simulink model "baseline_queso_1_1"  (R2021a)
settings: Solver=FixedStepAuto  StartTime=0.0  StopTime=50  FixedStep=framePeriod_s  RelTol=1e-3
undefined symbols (not defined in the file or in its folder): Aircraft, analog, aux, Earth, framePeriod_s, mode, motors_enabled, pwm, sbus, throttle_cmd_prcnt, waypoint_reached, WGS84
libraries: simulink x26, pid_lib x11, aerolibtransform2 x3, simulink_extras x2, aerolibguid x1
(part 1 of 3)
settings Model: Creator=brian  LastModifiedBy=Tuan Luong
settings SolverCC: AlgebraicLoopSolver=TrustRegion
settings OptimizationCC: DefaultParameterBehavior=Inlined  GainParamInheritBuiltInType=on  UseFloatMulNetSlope=on  DefaultUnderspecifiedDataType=single  InlineInvariantSignals=on  PassReuseOutputArgsAs=Individual arguments  ZeroExternalMemoryAtStartup=off  ZeroInternalMemoryAtStartup=off  NoFixptDivByZeroProtection=on  EfficientFloat2IntCast=on  LifeSpan=1  OptimizeBlockOrder=speed  DifferentSizesBufferReuse=on  EfficientTunableParamExpr=on
settings DebuggingCC: ParameterTunabilityLossMsg=error  SFMachineParentedDataDiag=warning
settings HardwareCC: ProdBitPerPointer=32  ProdBitPerSizeT=32  ProdBitPerPtrDiffT=32  ProdLargestAtomicInteger=Long  ProdLargestAtomicFloat=Double  ProdWordSize=32  ProdLongLongMode=on  ProdHWDeviceType=NXP->Cortex-M4
settings ModelReferenceCC: ModelReferenceNumInstancesAllowed=Single
settings SFSimCC: SimParseCustomCode=off  MATLABDynamicMemAlloc=off
settings RTWCC: SystemTargetFile=ert.tlc  GenCodeOnly=on  TemplateMakefile=ert_default_tmf  RTWVerbose=off  Toolchain=Microsoft Visual C++ 2019 v16.0 | nmake (64-bit Windows)  BuildConfiguration=Faster Runs  TargetLang=C++
settings CodeAppCC: ForceParamTrailComments=on  IgnoreCustomStorageClasses=off  OperatorAnnotations=on  SimulinkDataObjDesc=on  SFDataObjDesc=on  CustomSymbolStrGlobalVar=rt$N$M  CustomSymbolStrType=$N$M  CustomSymbolStrFcn=$N$M$F  CustomSymbolStrMacro=$N$M  InsertBlockDesc=on
settings ERTTargetCC: TargetLangStandard=C++03 (ISO)  IncludeMdlTerminateFcn=off  CombineSignalStateStructs=on  SuppressErrorStatus=on  SupportAbsoluteTime=off  CodeInterfacePackaging=C++ class  SupportNonFinite=off  SupportComplex=off  ERTHeaderFileRootName=autocode$E  ERTSourceFileRootName=autocode$E  InlinedParameterPlacement=NonHierarchical  RootIOFormat=Structure reference  ERTCustomFileTemplate=example_file_process.tlc  ERTFilePackagingFormat=Compact  ArrayContainerType=std::array

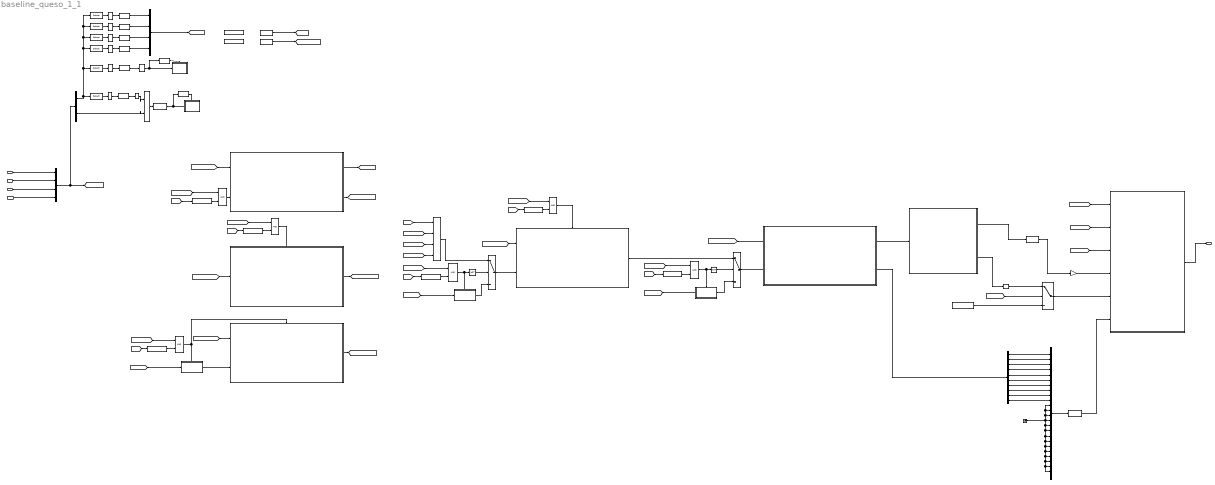
== system baseline_queso_1_1 ==
  System Data : Inport  OutDataTypeStr=Bus: SysData  SampleTime=framePeriod_s  BusOutputAsStruct=on
  Sensor Data : Inport  Port=2  OutDataTypeStr=Bus: SensorData  SampleTime=framePeriod_s  BusOutputAsStruct=on
  Navigation Filter Data : Inport  Port=3  OutDataTypeStr=Bus: NavData  SampleTime=framePeriod_s  BusOutputAsStruct=on
  Telemetry Data : Inport  Port=4  OutDataTypeStr=Bus: TelemData  SampleTime=framePeriod_s  BusOutputAsStruct=on
  ANGLE CONTROLLER : Subsystem
  Bus Creator2 : BusCreator  Inputs=24
  Bus Selector : BusSelector  OutputSignals=Sensor Data.inceptor.ch,Navigation Filter Data.nav_initialized
  Bus Selector1 : BusSelector  OutputSignals=throttle,roll_cc,roll_cmd_rad,roll_rad,pitch_cc,pitch_cmd_rad,pitch_rad,yaw_cc,yaw_rate_cmd_radps,yaw_rate_radps
  Cast To Boolean1 : DataTypeConversion  OutDataTypeStr=boolean
  Cast To Single : DataTypeConversion  OutDataTypeStr=single
  Cast To Single1 : DataTypeConversion  OutDataTypeStr=single
  Compare To Constant : simulink/Logic and Bit Operations/Compare To Constant  relop=>  const=0  OutDataTypeStr=boolean
  Constant : Constant  Value=[0 0 0 0 0 0 0 0]  OutDataTypeStr=single  SampleTime=framePeriod_s
  Data Store Read : DataStoreRead  DataStoreName=cur_mode  SampleTime=framePeriod_s  IndexOptions=Index vector (dialog)  Indices=1  OutputSizes=1
  Data Store Read1 : DataStoreRead  DataStoreName=motor_state  SampleTime=framePeriod_s  IndexOptions=Index vector (dialog)  Indices=1  OutputSizes=1
  Data Type Conversion{,1..5} (6 alike) : DataTypeConversion  OutDataTypeStr=single
  Data Type Conversion6 : DataTypeConversion  OutDataTypeStr=int8  RndMeth=Nearest
  Gain : Gain  Gain=100
  Ground : Ground
  LAND CONTROLLER : Subsystem
  Motor Mixing Algorithm : Subsystem
  Multiport Switch : MultiPortSwitch  DataPortOrder=Specify indices  DataPortIndices={2,3,4}  DiagnosticForDefault=None
  NOT : Logic  Operator=NOT  IconShape=distinctive  AllPortsSameDT=off  OutDataTypeStr=boolean
  NOT1 : Logic  Operator=NOT  IconShape=distinctive  AllPortsSameDT=off  OutDataTypeStr=boolean
  POS_HOLD CONTROLLER : Subsystem
  Pos_Hold_input_conversion : Subsystem
  Pos_Hold_input_conversion2 : Subsystem
  RTL CONTROLLER : Subsystem
  Reshape : Reshape
  Stab_input_conversion : Subsystem
  Switch : Switch  Criteria=u2 > Threshold  Threshold=0.5
  Switch1 : Switch  Criteria=u2 > Threshold  Threshold=0.5
  To VMS Data : Subsystem
  WAYPOINT CONTROLLER : Subsystem
  cmd_bus : BusCreator  Inputs=4
  compare_to_land : simulink/Logic and Bit Operations/Compare To Constant  relop===  const=4  OutDataTypeStr=boolean
  compare_to_pos_hold : simulink/Logic and Bit Operations/Compare To Constant  relop=>  const=0  OutDataTypeStr=boolean
  compare_to_rtl : simulink/Logic and Bit Operations/Compare To Constant  relop===  const=3  OutDataTypeStr=boolean
  compare_to_stab : simulink/Logic and Bit Operations/Compare To Constant  relop=<=  const=0  OutDataTypeStr=boolean
  compare_to_stab1 : simulink/Logic and Bit Operations/Compare To Constant  relop===  const=1  OutDataTypeStr=boolean
  compare_to_wp : simulink/Logic and Bit Operations/Compare To Constant  relop===  const=2  OutDataTypeStr=boolean
  data_sys_bus : BusCreator  Inputs=4
  detect_manual_arming : simulink/Logic and Bit Operations/Detect Change  vinit=0  OutDataTypeStr=boolean
  detect_mode_change : simulink/Logic and Bit Operations/Detect Change  vinit=0  OutDataTypeStr=boolean
  flight_mode : DataStoreMemory  DataStoreName=cur_mode  ReadBeforeWriteMsg=warning  WriteAfterWriteMsg=warning  WriteAfterReadMsg=warning  ShowAdditionalParam=off  OutDataTypeStr=int8
  manual_arming : Subsystem
  manual_mode_selection : Subsystem
  mode_norm : Polyval  Coefs=Aircraft.Inceptor.coef_3
  motor_armed AND mode_{0..5} (6 alike) : Logic  IconShape=distinctive  AllPortsSameDT=off  OutDataTypeStr=boolean
  motor_state : DataStoreMemory  DataStoreName=motor_state  ReadBeforeWriteMsg=warning  WriteAfterWriteMsg=warning  WriteAfterReadMsg=warning  ShowAdditionalParam=off  OutDataTypeStr=boolean
  nav_init AND motor_enable : Logic  IconShape=distinctive  AllPortsSameDT=off  OutDataTypeStr=boolean
  pitch_norm : Polyval  Coefs=Aircraft.Inceptor.coef_2
  roll_norm : Polyval  Coefs=Aircraft.Inceptor.coef_2
  select_mode : Selector  IndexOptions=Index vector (dialog)  Indices=Aircraft.Inceptor.mode0  OutputSizes=1
  select_pitch : Selector  IndexOptions=Index vector (dialog)  Indices=Aircraft.Inceptor.pitch  OutputSizes=1
  select_roll : Selector  IndexOptions=Index vector (dialog)  Indices=Aircraft.Inceptor.roll  OutputSizes=1
  select_throttle : Selector  IndexOptions=Index vector (dialog)  Indices=Aircraft.Inceptor.throttle  OutputSizes=1
  select_throttle_en : Selector  IndexOptions=Index vector (dialog)  Indices=Aircraft.Inceptor.throttle_en  OutputSizes=1
  select_yaw : Selector  IndexOptions=Index vector (dialog)  Indices=Aircraft.Inceptor.yaw  OutputSizes=1
  switch_motor_out : Switch  Criteria=u2 > Threshold
  throttle_en_norm : Polyval  Coefs=Aircraft.Inceptor.coef_2
  throttle_norm : Polyval  Coefs=Aircraft.Inceptor.coef_1
  yaw_norm : Polyval  Coefs=Aircraft.Inceptor.coef_2
  VmsData : Outport  OutDataTypeStr=Bus: VmsData  SampleTime=framePeriod_s  BusOutputAsStruct=on
  wires:
  Telemetry Data/1 -> data_sys_bus/3  "Telemetry Data"
  System Data/1 -> data_sys_bus/4  "System Data"
  Sensor Data/1 -> data_sys_bus/1  "Sensor Data"
  Navigation Filter Data/1 -> data_sys_bus/2  "Navigation Filter Data"
  To VMS Data/1(VmsData) -> VmsData/1  "VmsData"
  [arm_state] -> motor_armed AND mode_0/1
  [arm_state] -> motor_armed AND mode_1/1
  [Mode] -> compare_to_pos_hold/1
  compare_to_pos_hold/1 -> motor_armed AND mode_1/2
  Motor Mixing Algorithm/2(PWM) -> Reshape/1
  switch_motor_out/1 -> To VMS Data/5(PWM In)
  [arm_state] -> switch_motor_out/2
  Constant/1 -> switch_motor_out/3
  ANGLE CONTROLLER/1(Command out) -> Motor Mixing Algorithm/1(MMA Bus)
  compare_to_stab/1 -> motor_armed AND mode_0/2
  [Mode] -> compare_to_stab/1
  [Mode] -> To VMS Data/3(Mode in)
  compare_to_wp/1 -> motor_armed AND mode_2/2
  [Mode] -> compare_to_wp/1
  [arm_state] -> motor_armed AND mode_2/1
  Bus Selector/2 -> nav_init AND motor_enable/2  "<nav_initialized>"
  WAYPOINT CONTROLLER/2(wp_reached) -> [waypoint_reached]
  nav_init AND motor_enable/1 -> Cast To Boolean1/1
  [waypoint_reached] -> To VMS Data/2(waypoint_reached)
  [arm_state] -> To VMS Data/1(motors_enabled)
  Motor Mixing Algorithm/1(throttle) -> Cast To Single1/1
  Bus Selector/1 -> select_throttle/1, select_pitch/1, select_roll/1, select_yaw/1, select_mode/1, select_throttle_en/1  "<ch>"
  select_throttle/1 -> Data Type Conversion5/1
  select_pitch/1 -> Data Type Conversion4/1
  select_roll/1 -> Data Type Conversion3/1
  select_yaw/1 -> Data Type Conversion2/1
  select_mode/1 -> Data Type Conversion1/1
  throttle_norm/1 -> cmd_bus/1  "throttle"
  pitch_norm/1 -> cmd_bus/2  "pitch"
  roll_norm/1 -> cmd_bus/3  "roll"
  yaw_norm/1 -> cmd_bus/4  "yaw"
  throttle_en_norm/1 -> Compare To Constant/1  "throttle_en"
  Compare To Constant/1 -> nav_init AND motor_enable/1
  cmd_bus/1 -> [cmd]
  select_throttle_en/1 -> Data Type Conversion/1
  Data Type Conversion/1 -> throttle_en_norm/1
  Data Type Conversion1/1 -> mode_norm/1
  Data Type Conversion2/1 -> yaw_norm/1
  Data Type Conversion3/1 -> roll_norm/1
  Data Type Conversion4/1 -> pitch_norm/1
  Data Type Conversion5/1 -> throttle_norm/1
  mode_norm/1 -> Data Type Conversion6/1  "mode"
  Data Store Read/1 -> [Mode]
  Data Type Conversion6/1 -> manual_mode_selection/1(mode_input), detect_mode_change/1
  detect_mode_change/1 -> manual_mode_selection/Enable
  detect_manual_arming/1 -> manual_arming/Enable
  Cast To Boolean1/1 -> detect_manual_arming/1, manual_arming/1(mode_input)
  Data Store Read1/1 -> [arm_state]
  Pos_Hold_input_conversion2/1(pos_hold_input) -> LAND CONTROLLER/2(Cmd_input)
  compare_to_land/1 -> motor_armed AND mode_4/2
  data_sys_bus/1 -> [sys_input], Bus Selector/1
  [Mode] -> compare_to_land/1
  [arm_state] -> motor_armed AND mode_4/1
  [arm_state] -> motor_armed AND mode_3/1
  motor_armed AND mode_3/1 -> RTL CONTROLLER/Enable
  compare_to_rtl/1 -> motor_armed AND mode_3/2
  [Mode] -> compare_to_rtl/1
  Bus Creator2/1 -> Cast To Single/1
  Gain/1 -> To VMS Data/4(throttle_cmd_prcnt)
  Ground/1 -> Bus Creator2/20, Bus Creator2/21, Bus Creator2/24, Bus Creator2/23, Bus Creator2/22, Bus Creator2/19, Bus Creator2/18, Bus Creator2/17, Bus Creator2/16, Bus Creator2/15, Bus Creator2/11, Bus Creator2/12, Bus Creator2/13, Bus Creator2/14
  Cast To Single/1 -> To VMS Data/6(Aux)
  Cast To Single1/1 -> Gain/1
  [cmd] -> Stab_input_conversion/1(cmd)
  motor_armed AND mode_0/1 -> NOT/1, Stab_input_conversion/Enable
  [sys_input] -> ANGLE CONTROLLER/1(Sys_input)
  Switch/1 -> ANGLE CONTROLLER/2(Cmd_input)
  NOT/1 -> Switch/2
  Stab_input_conversion/1(angle_ctrl_input) -> Switch/3
  [sys_input] -> POS_HOLD CONTROLLER/1(Sys_input)
  motor_armed AND mode_1/1 -> POS_HOLD CONTROLLER/Enable
  [cmd] -> Pos_Hold_input_conversion/1(cmd)
  motor_armed AND mode_5/1 -> Pos_Hold_input_conversion/Enable, NOT1/1
  [Mode] -> compare_to_stab1/1
  compare_to_stab1/1 -> motor_armed AND mode_5/2
  [arm_state] -> motor_armed AND mode_5/1
  NOT1/1 -> Switch1/2
  Switch1/1 -> POS_HOLD CONTROLLER/2(Cmd_input)
  Pos_Hold_input_conversion/1(pos_hold_input) -> Switch1/3
  POS_HOLD CONTROLLER/1(Command out) -> Switch/1
  motor_armed AND mode_2/1 -> WAYPOINT CONTROLLER/2(auto_trigger)
  Multiport Switch/1 -> Switch1/1
  [Mode] -> Multiport Switch/1
  WAYPOINT CONTROLLER/1(wp_command) -> [wp_cmd]
  [wp_cmd] -> Multiport Switch/2
  [sys_input] -> WAYPOINT CONTROLLER/1(Sys_input)
  [sys_input] -> RTL CONTROLLER/1(Sys_input)
  RTL CONTROLLER/1(Command out) -> [rtl_cmd]
  [rtl_cmd] -> Multiport Switch/3
  [sys_input] -> LAND CONTROLLER/1(Sys_input)
  [cmd] -> Pos_Hold_input_conversion2/1(cmd)
  LAND CONTROLLER/1(land_cmd) -> [land_cmd]
  [land_cmd] -> Multiport Switch/4
  motor_armed AND mode_4/1 -> LAND CONTROLLER/Enable, Pos_Hold_input_conversion2/Enable
  ANGLE CONTROLLER/2(inner_loop_log) -> Bus Selector1/1
  Bus Selector1/1 -> Bus Creator2/1  "<throttle>"
  Bus Selector1/2 -> Bus Creator2/2  "<roll_cc>"
  Bus Selector1/3 -> Bus Creator2/3  "<roll_cmd_rad>"
  Bus Selector1/4 -> Bus Creator2/4  "<roll_rad>"
  Bus Selector1/5 -> Bus Creator2/5  "<pitch_cc>"
  Bus Selector1/6 -> Bus Creator2/6  "<pitch_cmd_rad>"
  Bus Selector1/8 -> Bus Creator2/8  "<yaw_cc>"
  Bus Selector1/7 -> Bus Creator2/7  "<pitch_rad>"
  Bus Selector1/9 -> Bus Creator2/9  "<yaw_rate_cmd_radps>"
  Bus Selector1/10 -> Bus Creator2/10  "<yaw_rate_radps>"
  Reshape/1 -> switch_motor_out/1

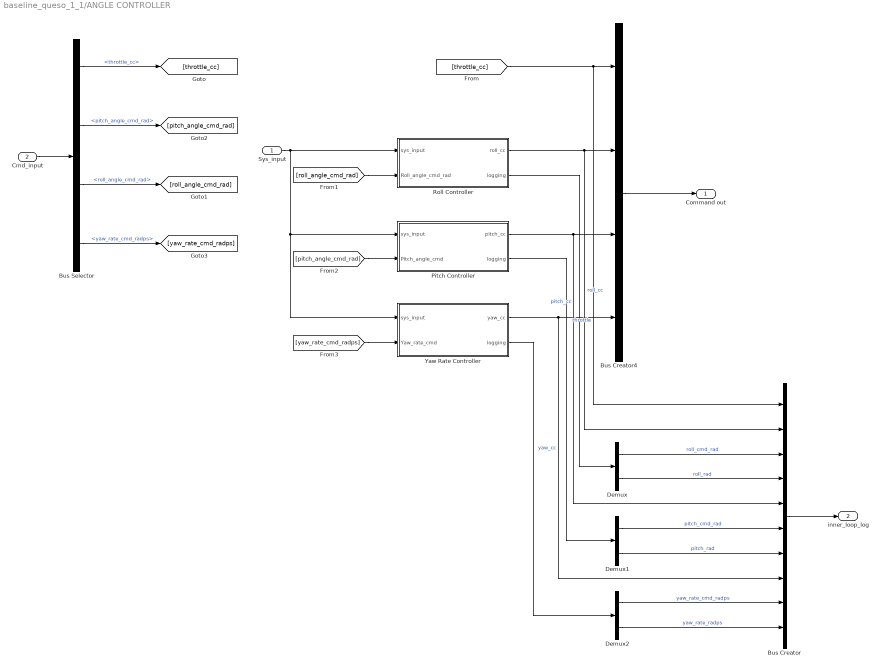
== system baseline_queso_1_1/ANGLE CONTROLLER ==
  Sys_input : Inport
  Cmd_input : Inport  Port=2
  Bus Creator : BusCreator  Inputs=10
  Bus Creator4 : BusCreator  Inputs=4
  Bus Selector : BusSelector  OutputSignals=throttle_cc,pitch_angle_cmd_rad,roll_angle_cmd_rad,yaw_rate_cmd_radps
  Demux : Demux  Outputs=2
  Demux1 : Demux  Outputs=2
  Demux2 : Demux  Outputs=2
  Pitch Controller : Subsystem
  Roll Controller : Subsystem
  Yaw Rate Controller : Subsystem
  Command out : Outport
  inner_loop_log : Outport  Port=2
  wires:
  Bus Creator4/1 -> Command out/1
  Cmd_input/1 -> Bus Selector/1
  Yaw Rate Controller/1(yaw_cc) -> Bus Creator4/4, Bus Creator/8  "yaw_cc"
  Pitch Controller/1(pitch_cc) -> Bus Creator4/3, Bus Creator/5  "pitch_cc"
  Roll Controller/1(roll_cc) -> Bus Creator4/2, Bus Creator/2  "roll_cc"
  Sys_input/1 -> Roll Controller/1(sys_input), Pitch Controller/1(sys_input), Yaw Rate Controller/1(sys_input)
  Bus Selector/1 -> [throttle_cc]  "<throttle_cc>"
  Bus Selector/4 -> [yaw_rate_cmd_radps]  "<yaw_rate_cmd_radps>"
  Bus Selector/2 -> [pitch_angle_cmd_rad]  "<pitch_angle_cmd_rad>"
  Bus Selector/3 -> [roll_angle_cmd_rad]  "<roll_angle_cmd_rad>"
  [throttle_cc] -> Bus Creator/1, Bus Creator4/1  "throttle"
  [roll_angle_cmd_rad] -> Roll Controller/2(Roll_angle_cmd_rad)
  [pitch_angle_cmd_rad] -> Pitch Controller/2(Pitch_angle_cmd)
  [yaw_rate_cmd_radps] -> Yaw Rate Controller/2(Yaw_rate_cmd)
  Demux/1 -> Bus Creator/3  "roll_cmd_rad"
  Demux/2 -> Bus Creator/4  "roll_rad"
  Roll Controller/2(logging) -> Demux/1
  Demux1/1 -> Bus Creator/6  "pitch_cmd_rad"
  Demux1/2 -> Bus Creator/7  "pitch_rad"
  Pitch Controller/2(logging) -> Demux1/1
  Demux2/1 -> Bus Creator/9  "yaw_rate_cmd_radps"
  Demux2/2 -> Bus Creator/10  "yaw_rate_radps"
  Yaw Rate Controller/2(logging) -> Demux2/1
  Bus Creator/1 -> inner_loop_log/1

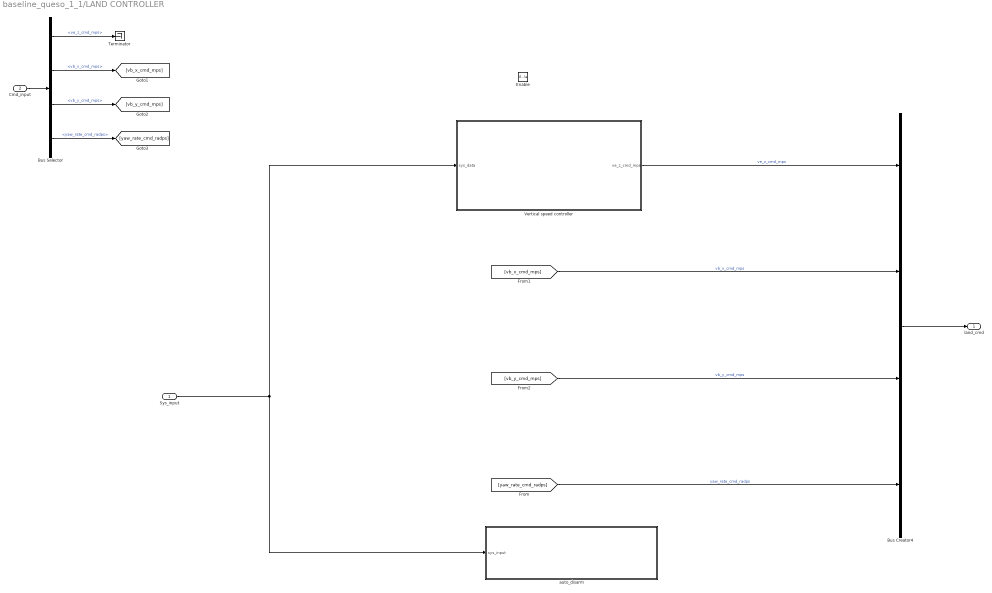
== system baseline_queso_1_1/LAND CONTROLLER ==
  Sys_input : Inport
  Cmd_input : Inport  Port=2
  Enable : EnablePort  PropagateVarSize=During execution
  Bus Creator4 : BusCreator  Inputs=4
  Bus Selector : BusSelector  OutputSignals=ve_z_cmd_mps,vb_x_cmd_mps,vb_y_cmd_mps,yaw_rate_cmd_radps
  Terminator : Terminator
  Vertical speed controller : Subsystem
  auto_disarm : Subsystem
  land_cmd : Outport
  wires:
  Bus Creator4/1 -> land_cmd/1
  Sys_input/1 -> Vertical speed controller/1(sys_data), auto_disarm/1(sys_input)
  Vertical speed controller/1(ve_z_cmd_mps) -> Bus Creator4/1  "ve_z_cmd_mps"
  [vb_x_cmd_mps] -> Bus Creator4/2  "vb_x_cmd_mps"
  [vb_y_cmd_mps] -> Bus Creator4/3  "vb_y_cmd_mps"
  [yaw_rate_cmd_radps] -> Bus Creator4/4  "yaw_rate_cmd_radps"
  Cmd_input/1 -> Bus Selector/1
  Bus Selector/2 -> [vb_x_cmd_mps]  "<vb_x_cmd_mps>"
  Bus Selector/4 -> [yaw_rate_cmd_radps]  "<yaw_rate_cmd_radps>"
  Bus Selector/3 -> [vb_y_cmd_mps]  "<vb_y_cmd_mps>"
  Bus Selector/1 -> Terminator/1  "<ve_z_cmd_mps>"

== system baseline_queso_1_1/Motor Mixing Algorithm ==
  MMA Bus : Inport
  Bus Selector : BusSelector  OutputSignals=throttle,roll_cc,pitch_cc,yaw_cc
  Motor Mix : Constant  Value=Aircraft.Motor.mix  OutDataTypeStr=single  SampleTime=framePeriod_s
  Multiply : Product  Inputs=**  Multiplication=Matrix(*)  OutDataTypeStr=single
  Mux : Mux
  Reshape : Reshape  OutputDimensionality=Column vector (2-D)
  Saturation : Saturate  UpperLimit=3000  LowerLimit=Aircraft.Control.motor_spin_min
  throttle : Outport
  PWM : Outport  Port=2
  wires:
  Mux/1 -> Reshape/1
  MMA Bus/1 -> Bus Selector/1
  Bus Selector/1 -> throttle/1, Mux/1  "<throttle>"
  Bus Selector/2 -> Mux/2  "<roll_cc>"
  Bus Selector/3 -> Mux/3  "<pitch_cc>"
  Bus Selector/4 -> Mux/4  "<yaw_cc>"
  Multiply/1 -> Saturation/1  "Command"
  Saturation/1 -> PWM/1
  Reshape/1 -> Multiply/2
  Motor Mix/1 -> Multiply/1

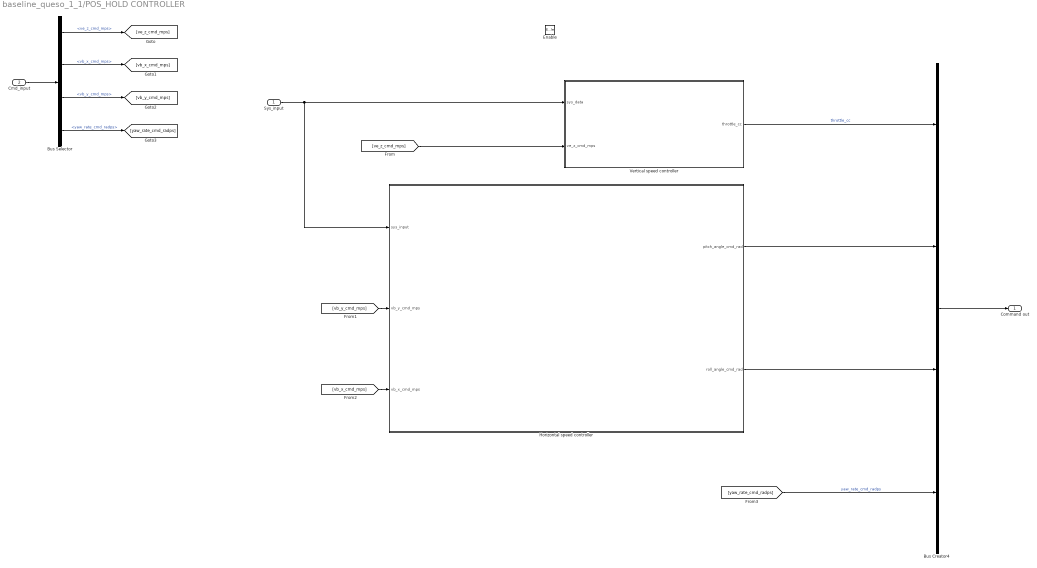
== system baseline_queso_1_1/POS_HOLD CONTROLLER ==
  Sys_input : Inport
  Cmd_input : Inport  Port=2
  Enable : EnablePort  PropagateVarSize=During execution
  Bus Creator4 : BusCreator  Inputs=4
  Bus Selector : BusSelector  OutputSignals=ve_z_cmd_mps,vb_x_cmd_mps,vb_y_cmd_mps,yaw_rate_cmd_radps
  Horizontal speed controller : Subsystem
  Vertical speed controller : Subsystem
  Command out : Outport
  wires:
  Bus Creator4/1 -> Command out/1
  Vertical speed controller/1(throttle_cc) -> Bus Creator4/1  "throttle_cc"
  Sys_input/1 -> Horizontal speed controller/1(sys_input), Vertical speed controller/1(sys_data)
  Cmd_input/1 -> Bus Selector/1
  Bus Selector/1 -> [ve_z_cmd_mps]  "<ve_z_cmd_mps>"
  Bus Selector/2 -> [vb_x_cmd_mps]  "<vb_x_cmd_mps>"
  Bus Selector/3 -> [vb_y_cmd_mps]  "<vb_y_cmd_mps>"
  Bus Selector/4 -> [yaw_rate_cmd_radps]  "<yaw_rate_cmd_radps>"
  [yaw_rate_cmd_radps] -> Bus Creator4/4  "yaw_rate_cmd_radps"
  [ve_z_cmd_mps] -> Vertical speed controller/2(ve_z_cmd_mps)
  [vb_y_cmd_mps] -> Horizontal speed controller/2(vb_y_cmd_mps)
  [vb_x_cmd_mps] -> Horizontal speed controller/3(vb_x_cmd_mps)
  Horizontal speed controller/1(pitch_angle_cmd_rad) -> Bus Creator4/2
  Horizontal speed controller/2(roll_angle_cmd_rad) -> Bus Creator4/3

== system baseline_queso_1_1/Pos_Hold_input_conversion ==
  cmd : Inport
  Enable : EnablePort
  Bus Creator : BusCreator  Inputs=4
  Bus Selector2 : BusSelector  OutputSignals=throttle,pitch,roll,yaw
  Gain1 : Gain  Gain=Aircraft.Control.v_hor_max
  Gain2 : Gain  Gain=Aircraft.Control.v_hor_max
  Gain3 : Gain  Gain=Aircraft.Control.yaw_rate_max
  Throttle Mapper : Subsystem
  pos_hold_input : Outport
  wires:
  Bus Selector2/3 -> Gain2/1  "<roll>"
  Gain2/1 -> Bus Creator/3  "vb_y_cmd_mps"
  Bus Selector2/1 -> Throttle Mapper/1(Throttle)  "<throttle>"
  Bus Selector2/2 -> Gain1/1  "<pitch>"
  Bus Creator/1 -> pos_hold_input/1  "pos_hold_input"
  Bus Selector2/4 -> Gain3/1  "<yaw>"
  Gain1/1 -> Bus Creator/2  "vb_x_cmd_mps"
  Gain3/1 -> Bus Creator/4  "yaw_rate_cmd_radps"
  cmd/1 -> Bus Selector2/1
  Throttle Mapper/1(Relative Velocity) -> Bus Creator/1  "ve_z_cmd_mps"

== system baseline_queso_1_1/Pos_Hold_input_conversion2 ==
  cmd : Inport
  Enable : EnablePort
  Bus Creator : BusCreator  Inputs=4
  Bus Selector2 : BusSelector  OutputSignals=throttle,pitch,roll,yaw
  Gain1 : Gain  Gain=Aircraft.Control.v_hor_max
  Gain2 : Gain  Gain=Aircraft.Control.v_hor_max
  Gain3 : Gain  Gain=Aircraft.Control.yaw_rate_max
  Throttle Mapper : Subsystem
  pos_hold_input : Outport
  wires:
  Bus Selector2/3 -> Gain2/1  "<roll>"
  Gain2/1 -> Bus Creator/3  "vb_y_cmd_mps"
  Bus Selector2/1 -> Throttle Mapper/1(Throttle)  "<throttle>"
  Bus Selector2/2 -> Gain1/1  "<pitch>"
  Bus Creator/1 -> pos_hold_input/1  "pos_hold_input"
  Bus Selector2/4 -> Gain3/1  "<yaw>"
  Gain1/1 -> Bus Creator/2  "vb_x_cmd_mps"
  Gain3/1 -> Bus Creator/4  "yaw_rate_cmd_radps"
  cmd/1 -> Bus Selector2/1
  Throttle Mapper/1(Relative Velocity) -> Bus Creator/1  "ve_z_cmd_mps"

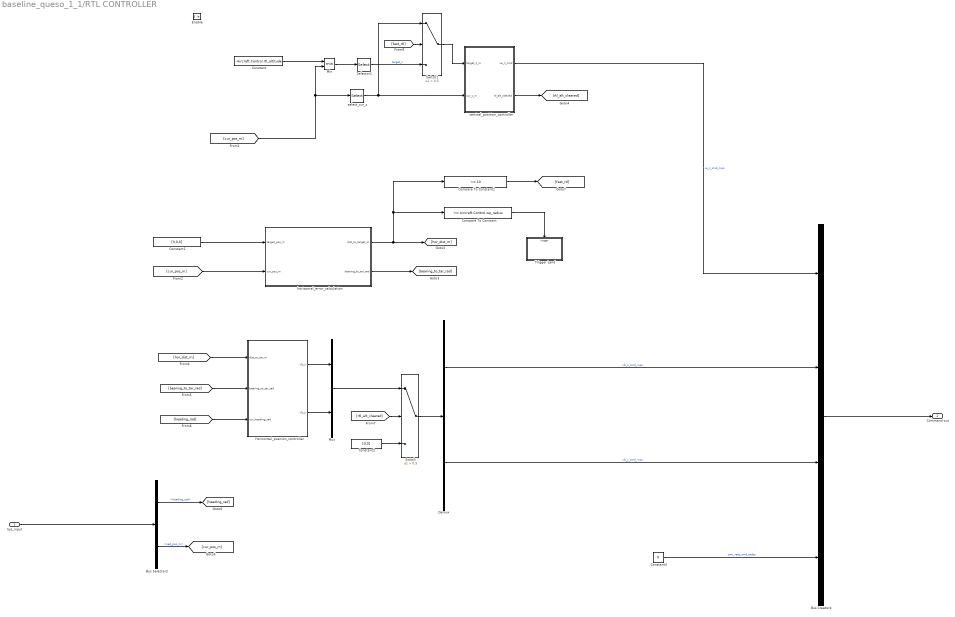
== system baseline_queso_1_1/RTL CONTROLLER ==
  Sys_input : Inport
  Enable : EnablePort
  Bus Creator4 : BusCreator  Inputs=4
  Bus Selector2 : BusSelector  OutputSignals=Navigation Filter Data.heading_rad,Navigation Filter Data.ned_pos_m
  Compare To Constant : simulink/Logic and Bit Operations/Compare To Constant  relop=<=  const=Aircraft.Control.wp_radius  OutDataTypeStr=boolean
  Compare To Constant1 : simulink/Logic and Bit Operations/Compare To Constant  relop=<=  const=10  OutDataTypeStr=boolean
  Constant : Constant  Value=-Aircraft.Control.rtl_altitude  OutDataTypeStr=single  SampleTime=-1
  Constant1 : Constant  Value=[0,0,0]  OutDataTypeStr=single  SampleTime=-1
  Constant2 : Constant  Value=[0,0]  OutDataTypeStr=single  SampleTime=-1
  Constant3 : Constant  Value=0  OutDataTypeStr=single  SampleTime=-1
  Demux : Demux  Outputs=2
  Horizontal_position_controller : Subsystem
  Min : MinMax  Inputs=2
  Mux : Mux  Inputs=2
  Selector1 : Selector  InputPortWidth=3  IndexOptions=Index vector (dialog)  Indices=3  OutputSizes=1
  Switch : Switch  Criteria=u2 > Threshold  Threshold=0.5
  Switch1 : Switch  Criteria=u2 > Threshold  Threshold=0.5
  Trigger Land : Subsystem
  "horizontal_error_calculation " : Subsystem
  select_cur_z : Selector  InputPortWidth=3  IndexOptions=Index vector (dialog)  Indices=3  OutputSizes=1
  vertical_position_controller : Subsystem
  Command out : Outport
  wires:
  Demux/2 -> Bus Creator4/3  "vb_y_cmd_mps"
  Demux/1 -> Bus Creator4/2  "vb_x_cmd_mps"
  Constant3/1 -> Bus Creator4/4  "yaw_rate_cmd_radps"
  vertical_position_controller/1(ve_z_cmd) -> Bus Creator4/1  "ve_z_cmd_mps"
  Bus Creator4/1 -> Command out/1
  Min/1 -> Selector1/1
  Constant/1 -> Min/1
  select_cur_z/1 -> vertical_position_controller/2(cur_z_m), Switch1/1
  [cur_pos_m] -> Min/2, select_cur_z/1
  Compare To Constant/1 -> Trigger Land/Trigger
  "horizontal_error_calculation "/2(bearing_to_tar_rad) -> [bearing_to_tar_rad]
  "horizontal_error_calculation "/1(dist_to_target_m) -> Compare To Constant/1, Compare To Constant1/1, [hor_dist_m]
  [cur_pos_m] -> "horizontal_error_calculation "/2(cur_pos_m)
  Constant1/1 -> "horizontal_error_calculation "/1(target_pos_m)
  [heading_rad] -> Horizontal_position_controller/3(cur_heading_rad)
  [bearing_to_tar_rad] -> Horizontal_position_controller/2(bearing_to_tar_rad)
  [hor_dist_m] -> Horizontal_position_controller/1(dist_to_tar_m)
  Sys_input/1 -> Bus Selector2/1
  Bus Selector2/1 -> [heading_rad]  "<heading_rad>"
  Bus Selector2/2 -> [cur_pos_m]  "<ned_pos_m>"
  vertical_position_controller/2(rtl_alt_cleared) -> [rtl_alt_cleared]
  Horizontal_position_controller/1(vb_x) -> Mux/1
  Horizontal_position_controller/2(vb_y) -> Mux/2
  Switch/1 -> Demux/1
  [rtl_alt_cleared] -> Switch/2
  Mux/1 -> Switch/1
  Constant2/1 -> Switch/3
  Compare To Constant1/1 -> [fast_rtl]
  Selector1/1 -> Switch1/3  "target_z"
  [fast_rtl] -> Switch1/2
  Switch1/1 -> vertical_position_controller/1(target_z_m)

== system baseline_queso_1_1/Stab_input_conversion ==
  cmd : Inport
  Enable : EnablePort
  Bus Creator : BusCreator  Inputs=4
  Bus Selector2 : BusSelector  OutputSignals=throttle,pitch,roll,yaw
  Gain : Gain
  Gain1 : Gain  Gain=-Aircraft.Control.pitch_angle_lim
  Gain2 : Gain  Gain=Aircraft.Control.roll_angle_lim
  Gain3 : Gain  Gain=Aircraft.Control.yaw_rate_max
  angle_ctrl_input : Outport
  wires:
  Bus Selector2/3 -> Gain2/1  "<roll>"
  Gain2/1 -> Bus Creator/3  "roll_angle_cmd_rad"
  Bus Selector2/2 -> Gain1/1  "<pitch>"
  Bus Creator/1 -> angle_ctrl_input/1  "angle_ctrl_input"
  Bus Selector2/4 -> Gain3/1  "<yaw>"
  Gain1/1 -> Bus Creator/2  "pitch_angle_cmd_rad"
  Gain3/1 -> Bus Creator/4  "yaw_rate_cmd_radps"
  cmd/1 -> Bus Selector2/1
  Bus Selector2/1 -> Gain/1  "<throttle>"
  Gain/1 -> Bus Creator/1  "throttle_cc"

== system baseline_queso_1_1/To VMS Data ==
  motors_enabled : Inport
  waypoint_reached : Inport  Port=2
  Mode in : Inport  Port=3
  throttle_cmd_prcnt : Inport  Port=4
  PWM In : Inport  Port=5
  Aux : Inport  Port=6
  Bus Creator : BusCreator  Inputs=motors_enabled,waypoint_reached,mode,throttle_cmd_prcnt,aux,sbus,pwm,analog  OutDataTypeStr=Bus: VmsData  NonVirtualBus=on
  Bus Creator1 : BusCreator  Inputs=1  OutDataTypeStr=Bus: AnalogData
  Ground : Ground
  SBUS & AUX1 : Subsystem
  Subsystem : Subsystem
  VmsData : Outport
  wires:
  waypoint_reached/1 -> Bus Creator/2  "waypoint_reached"
  Mode in/1 -> Bus Creator/3  "mode"
  motors_enabled/1 -> Bus Creator/1  "motors_enabled"
  Bus Creator/1 -> VmsData/1
  throttle_cmd_prcnt/1 -> Bus Creator/4  "throttle_cmd_prcnt"
  PWM In/1 -> Subsystem/1(norm_pwm)  "pwm"
  Subsystem/1(PwmCmd) -> Bus Creator/7  "pwm"
  Bus Creator1/1 -> Bus Creator/8  "analog"
  Ground/1 -> Bus Creator1/1  "val"
  Aux/1 -> Bus Creator/5  "aux"
  SBUS & AUX1/1(sbus) -> Bus Creator/6  "sbus"

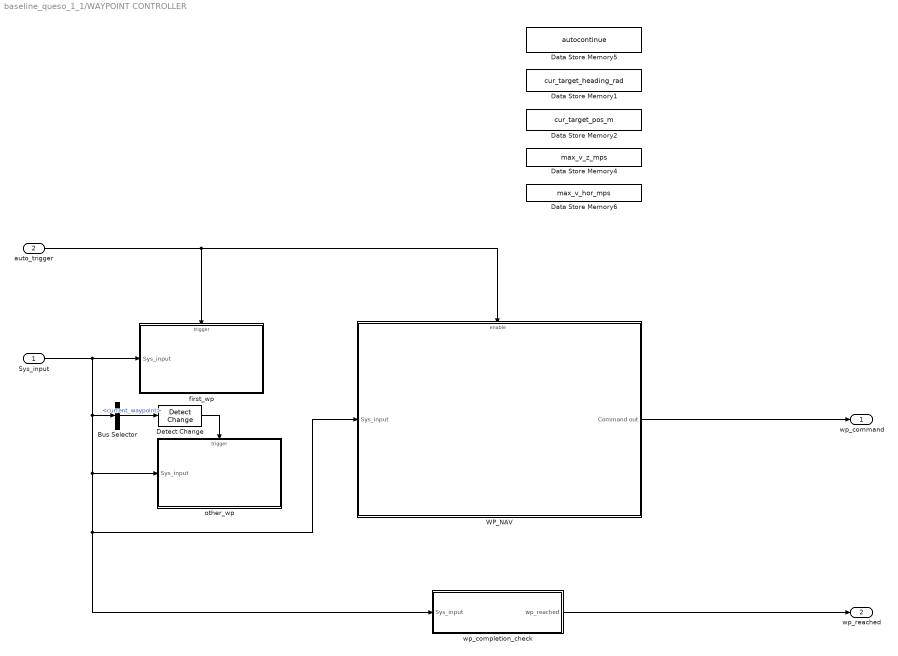
== system baseline_queso_1_1/WAYPOINT CONTROLLER ==
  Sys_input : Inport
  auto_trigger : Inport  Port=2
  Bus Selector : BusSelector  OutputSignals=Telemetry Data.current_waypoint
  Data Store Memory1 : DataStoreMemory  DataStoreName=cur_target_heading_rad  ReadBeforeWriteMsg=warning  WriteAfterWriteMsg=warning  WriteAfterReadMsg=warning  ShowAdditionalParam=off  OutDataTypeStr=single
  Data Store Memory2 : DataStoreMemory  DataStoreName=cur_target_pos_m  ReadBeforeWriteMsg=warning  WriteAfterWriteMsg=warning  WriteAfterReadMsg=warning  InitialValue=[10 10 10]  ShowAdditionalParam=off  OutDataTypeStr=single
  Data Store Memory4 : DataStoreMemory  DataStoreName=max_v_z_mps  ReadBeforeWriteMsg=warning  WriteAfterWriteMsg=warning  WriteAfterReadMsg=warning  ShowAdditionalParam=off  OutDataTypeStr=single
  Data Store Memory5 : DataStoreMemory  DataStoreName=autocontinue  ReadBeforeWriteMsg=warning  WriteAfterWriteMsg=warning  WriteAfterReadMsg=warning  InitialValue=1  ShowAdditionalParam=off  OutDataTypeStr=boolean
  Data Store Memory6 : DataStoreMemory  DataStoreName=max_v_hor_mps  ReadBeforeWriteMsg=warning  WriteAfterWriteMsg=warning  WriteAfterReadMsg=warning  ShowAdditionalParam=off  OutDataTypeStr=single
  Detect Change : simulink/Logic and Bit Operations/Detect Change  vinit=0  OutDataTypeStr=boolean
  WP_NAV : Subsystem
  first_wp : Subsystem  TreatAsAtomicUnit=on
  other_wp : Subsystem  TreatAsAtomicUnit=on
  wp_completion_check : Subsystem
  wp_command : Outport
  wp_reached : Outport  Port=2
  wires:
  Sys_input/1 -> first_wp/1(Sys_input), WP_NAV/1(Sys_input), wp_completion_check/1(Sys_input), other_wp/1(Sys_input), Bus Selector/1
  auto_trigger/1 -> first_wp/Trigger, WP_NAV/Enable
  wp_completion_check/1(wp_reached) -> wp_reached/1
  Detect Change/1 -> other_wp/Trigger
  Bus Selector/1 -> Detect Change/1  "<current_waypoint>"
  WP_NAV/1(Command out) -> wp_command/1

== system baseline_queso_1_1/manual_arming ==
  mode_input : Inport
  Enable : EnablePort
  Data Store Write : DataStoreWrite  DataStoreName=motor_state  SampleTime=framePeriod_s  IndexOptions=Index vector (dialog)  Indices=1  OutputSizes=1
  wires:
  mode_input/1 -> Data Store Write/1

== system baseline_queso_1_1/manual_mode_selection ==
  mode_input : Inport
  Enable : EnablePort
  Data Store Write : DataStoreWrite  DataStoreName=cur_mode  SampleTime=framePeriod_s  IndexOptions=Index vector (dialog)  Indices=1  OutputSizes=1
  wires:
  mode_input/1 -> Data Store Write/1

== system baseline_queso_1_1/ANGLE CONTROLLER/Pitch Controller ==
  sys_input : Inport
  Pitch_angle_cmd : Inport  Port=2
  Bus Selector : BusSelector  OutputSignals=Navigation Filter Data.pitch_rad,Telemetry Data.param
  Demux : Demux  Outputs=3
  Mux : Mux  Inputs=2
  Selector : Selector  IndexMode=Zero-based  IndexOptions=Index vector (dialog)  Indices=[3 4 5]  OutputSizes=1
  stab_pitch_PID : pid_lib/PID Controller  Controller=PID  Form=Parallel  TimeDomain=Discrete-time  UseExternalTs=off  SampleTime=framePeriod_s  IntegratorMethod=Forward Euler  FilterMethod=Forward Euler  ControllerParametersSource=external  P=0.335  I=0.005  D=0  UseFilter=off  N=100  TunerSelectOption=Transfer Function Based (PID Tuner App)  InitialConditionSource=internal  InitialConditionForIntegrator=0  InitialConditionForFilter=0  DifferentiatorICPrevScaledInput=0  ExternalReset=none  TrackingMode=off  Kt=1  LimitOutput=off  SatLimitsSource=internal  UpperSaturationLimit=inf  LowerSaturationLimit=-inf  LinearizeAsGain=on  AntiWindupMode=clamping  Kb=1  POutMin=[]  POutMax=[]  IOutMin=[]  IOutMax=[]  DOutMin=[]  DOutMax=[]  NOutMin=[]  NOutMax=[]  SumOutMin=[]  SumOutMax=[]  SaturationOutMin=[]  SaturationOutMax=[]  PParamMin=[]  PParamMax=[]  IParamMin=[]  IParamMax=[]  DParamMin=[]  DParamMax=[]  NParamMin=[]  NParamMax=[]  KbParamMin=[]  KbParamMax=[]  KtParamMin=[]  KtParamMax=[]  KbOutMin=[]  KbOutMax=[]  KtOutMin=[]  KtOutMax=[]  IntegratorOutMin=[]  IntegratorOutMax=[]  FilterOutMin=[]  FilterOutMax=[]  SumI1OutMin=[]  SumI1OutMax=[]  SumI2OutMin=[]  SumI2OutMax=[]  SumI3OutMin=[]  SumI3OutMax=[]  SumI4OutMin=[]  SumI4OutMax=[]  SumDOutMin=[]  SumDOutMax=[]  DifferentiatorOutMin=[]  DifferentiatorOutMax=[]  FilterDiffOutCoefMin=[]  FilterDiffOutCoefMax=[]  ReciprocalOutMin=[]  ReciprocalOutMax=[]  SumDenOutMin=[]  SumDenOutMax=[]  SumNumOutMin=[]  SumNumOutMax=[]  DivideOutMin=[]  DivideOutMax=[]  UdiffTsProdOutMin=[]  UdiffTsProdOutMax=[]  NTsProdOutMin=[]  NTsProdOutMax=[]  UintegralTsProdOutMin=[]  UintegralTsProdOutMax=[]  UngainTsProdOutMin=[]  UngainTsProdOutMax=[]  IntegratorContinuousStateAttributes=''  IntegratorStateMustResolveToSignalObject=off  IntegratorRTWStateStorageClass=Auto  FilterContinuousStateAttributes=''  FilterStateMustResolveToSignalObject=off  FilterRTWStateStorageClass=Auto  ParallelPVariant=ExternalParameters  IdealPVariant=Disabled  IVariant=ExternalParameters  DVariant=ExternalParameters  IntegratorVariant=Discrete  SatVariant=Disabled  AWVariant=Passthrough  PCopyVariant=Disabled  TRVariant=Disabled  FdbkBlocksVariant=Forward  IdealPFdbkVariant=Disabled  SatFdbkVariant=Disabled  DerivativeFilterVariant=Differentiator  NVariant=Passthrough  NCopyVariant=Disabled_SignalSpec  FilterICVariant=InternalICsDifferentiator  IntegratorICVariant=InternalICs  ExternalResetVariant=Disabled  TRSumVariant=Passthrough  SumFdbkVariant=Disabled  SumVariant=Sum_PID  TsampFilterVariant=InternalTs  TsampNgainVariant=Passthrough  TsampIntegralVariant=Passthrough  ExternalSaturationOutDataTypeStr=Inherit: Same as second input
  stab_pitch_angle_error_calc : Sum  Inputs=|+-
  stab_pitch_rate_saturation : Saturate  UpperLimit=Aircraft.Control.pitch_rate_max  LowerLimit=-Aircraft.Control.pitch_rate_max  LinearizeAsGain=off
  pitch_cc : Outport
  logging : Outport  Port=2
  wires:
  stab_pitch_angle_error_calc/1 -> stab_pitch_PID/1  "pitch error"
  sys_input/1 -> Bus Selector/1
  Bus Selector/1 -> stab_pitch_angle_error_calc/2, Mux/2  "<pitch_rad>"
  Pitch_angle_cmd/1 -> Mux/1, stab_pitch_angle_error_calc/1  "pitch angle cmd"
  stab_pitch_PID/1 -> stab_pitch_rate_saturation/1
  Demux/3 -> stab_pitch_PID/4  "D_gain"
  Demux/2 -> stab_pitch_PID/3  "I_gain"
  Demux/1 -> stab_pitch_PID/2  "P_gain"
  stab_pitch_rate_saturation/1 -> pitch_cc/1
  Mux/1 -> logging/1
  Bus Selector/2 -> Selector/1  "<param>"
  Selector/1 -> Demux/1

== system baseline_queso_1_1/ANGLE CONTROLLER/Roll Controller ==
  sys_input : Inport
  Roll_angle_cmd_rad : Inport  Port=2
  Bus Selector : BusSelector  OutputSignals=Navigation Filter Data.roll_rad,Telemetry Data.param
  Demux : Demux  Outputs=3
  Mux : Mux  Inputs=2
  Selector : Selector  IndexMode=Zero-based  IndexOptions=Index vector (dialog)  Indices=[0 1 2]  OutputSizes=1
  stab_roll_PID : pid_lib/PID Controller  Controller=PID  Form=Parallel  TimeDomain=Discrete-time  UseExternalTs=off  SampleTime=framePeriod_s  IntegratorMethod=Forward Euler  FilterMethod=Forward Euler  ControllerParametersSource=external  P=0.335  I=0.005  D=0  UseFilter=off  N=100  TunerSelectOption=Transfer Function Based (PID Tuner App)  InitialConditionSource=internal  InitialConditionForIntegrator=0  InitialConditionForFilter=0  DifferentiatorICPrevScaledInput=0  ExternalReset=none  TrackingMode=off  Kt=1  LimitOutput=off  SatLimitsSource=internal  UpperSaturationLimit=inf  LowerSaturationLimit=-inf  LinearizeAsGain=on  AntiWindupMode=clamping  Kb=1  POutMin=[]  POutMax=[]  IOutMin=[]  IOutMax=[]  DOutMin=[]  DOutMax=[]  NOutMin=[]  NOutMax=[]  SumOutMin=[]  SumOutMax=[]  SaturationOutMin=[]  SaturationOutMax=[]  PParamMin=[]  PParamMax=[]  IParamMin=[]  IParamMax=[]  DParamMin=[]  DParamMax=[]  NParamMin=[]  NParamMax=[]  KbParamMin=[]  KbParamMax=[]  KtParamMin=[]  KtParamMax=[]  KbOutMin=[]  KbOutMax=[]  KtOutMin=[]  KtOutMax=[]  IntegratorOutMin=[]  IntegratorOutMax=[]  FilterOutMin=[]  FilterOutMax=[]  SumI1OutMin=[]  SumI1OutMax=[]  SumI2OutMin=[]  SumI2OutMax=[]  SumI3OutMin=[]  SumI3OutMax=[]  SumI4OutMin=[]  SumI4OutMax=[]  SumDOutMin=[]  SumDOutMax=[]  DifferentiatorOutMin=[]  DifferentiatorOutMax=[]  FilterDiffOutCoefMin=[]  FilterDiffOutCoefMax=[]  ReciprocalOutMin=[]  ReciprocalOutMax=[]  SumDenOutMin=[]  SumDenOutMax=[]  SumNumOutMin=[]  SumNumOutMax=[]  DivideOutMin=[]  DivideOutMax=[]  UdiffTsProdOutMin=[]  UdiffTsProdOutMax=[]  NTsProdOutMin=[]  NTsProdOutMax=[]  UintegralTsProdOutMin=[]  UintegralTsProdOutMax=[]  UngainTsProdOutMin=[]  UngainTsProdOutMax=[]  IntegratorContinuousStateAttributes=''  IntegratorStateMustResolveToSignalObject=off  IntegratorRTWStateStorageClass=Auto  FilterContinuousStateAttributes=''  FilterStateMustResolveToSignalObject=off  FilterRTWStateStorageClass=Auto  ParallelPVariant=ExternalParameters  IdealPVariant=Disabled  IVariant=ExternalParameters  DVariant=ExternalParameters  IntegratorVariant=Discrete  SatVariant=Disabled  AWVariant=Passthrough  PCopyVariant=Disabled  TRVariant=Disabled  FdbkBlocksVariant=Forward  IdealPFdbkVariant=Disabled  SatFdbkVariant=Disabled  DerivativeFilterVariant=Differentiator  NVariant=Passthrough  NCopyVariant=Disabled_SignalSpec  FilterICVariant=InternalICsDifferentiator  IntegratorICVariant=InternalICs  ExternalResetVariant=Disabled  TRSumVariant=Passthrough  SumFdbkVariant=Disabled  SumVariant=Sum_PID  TsampFilterVariant=InternalTs  TsampNgainVariant=Passthrough  TsampIntegralVariant=Passthrough  ExternalSaturationOutDataTypeStr=Inherit: Same as second input
  stab_roll_angle_error_calc : Sum  Inputs=|+-
  stab_roll_rate_saturation : Saturate  UpperLimit=Aircraft.Control.roll_rate_max  LowerLimit=-Aircraft.Control.roll_rate_max
  roll_cc : Outport
  logging : Outport  Port=2
  wires:
  stab_roll_PID/1 -> stab_roll_rate_saturation/1  "Roll_cmd"
  Roll_angle_cmd_rad/1 -> Mux/1, stab_roll_angle_error_calc/1  "roll_angle_command"
  stab_roll_angle_error_calc/1 -> stab_roll_PID/1  "roll_angle_error"
  sys_input/1 -> Bus Selector/1
  Bus Selector/1 -> stab_roll_angle_error_calc/2, Mux/2  "<roll_rad>"
  Demux/1 -> stab_roll_PID/2  "P_gain"
  Demux/2 -> stab_roll_PID/3  "I_gain"
  Demux/3 -> stab_roll_PID/4  "D_gain"
  stab_roll_rate_saturation/1 -> roll_cc/1
  Mux/1 -> logging/1
  Bus Selector/2 -> Selector/1  "<param>"
  Selector/1 -> Demux/1

== system baseline_queso_1_1/ANGLE CONTROLLER/Yaw Rate Controller ==
  sys_input : Inport
  Yaw_rate_cmd : Inport  Port=2
  Bus Selector : BusSelector  OutputSignals=Navigation Filter Data.gyro_radps,Telemetry Data.param
  Demux : Demux  Outputs=3
  Mux : Mux  Inputs=2
  Saturation : Saturate  UpperLimit=Aircraft.Control.yaw_rate_max  LowerLimit=-Aircraft.Control.yaw_rate_max  OutDataTypeStr=single
  Selector : Selector  InputPortWidth=3  IndexOptions=Index vector (dialog)  Indices=3  OutputSizes=1
  Selector1 : Selector  IndexMode=Zero-based  IndexOptions=Index vector (dialog)  Indices=[6 7 8]  OutputSizes=1
  stab_yaw_rate_PID : pid_lib/PID Controller  Controller=PID  Form=Parallel  TimeDomain=Discrete-time  UseExternalTs=off  SampleTime=framePeriod_s  IntegratorMethod=Forward Euler  FilterMethod=Forward Euler  ControllerParametersSource=external  P=1.85  I=0.01  D=0  UseFilter=off  N=100  TunerSelectOption=Transfer Function Based (PID Tuner App)  InitialConditionSource=internal  InitialConditionForIntegrator=0  InitialConditionForFilter=0  DifferentiatorICPrevScaledInput=0  ExternalReset=none  TrackingMode=off  Kt=1  LimitOutput=off  SatLimitsSource=internal  UpperSaturationLimit=inf  LowerSaturationLimit=-inf  LinearizeAsGain=off  AntiWindupMode=clamping  Kb=1  POutMin=[]  POutMax=[]  IOutMin=[]  IOutMax=[]  DOutMin=[]  DOutMax=[]  NOutMin=[]  NOutMax=[]  SumOutMin=[]  SumOutMax=[]  SaturationOutMin=[]  SaturationOutMax=[]  PParamMin=[]  PParamMax=[]  IParamMin=[]  IParamMax=[]  DParamMin=[]  DParamMax=[]  NParamMin=[]  NParamMax=[]  KbParamMin=[]  KbParamMax=[]  KtParamMin=[]  KtParamMax=[]  KbOutMin=[]  KbOutMax=[]  KtOutMin=[]  KtOutMax=[]  IntegratorOutMin=[]  IntegratorOutMax=[]  FilterOutMin=[]  FilterOutMax=[]  SumI1OutMin=[]  SumI1OutMax=[]  SumI2OutMin=[]  SumI2OutMax=[]  SumI3OutMin=[]  SumI3OutMax=[]  SumI4OutMin=[]  SumI4OutMax=[]  SumDOutMin=[]  SumDOutMax=[]  DifferentiatorOutMin=[]  DifferentiatorOutMax=[]  FilterDiffOutCoefMin=[]  FilterDiffOutCoefMax=[]  ReciprocalOutMin=[]  ReciprocalOutMax=[]  SumDenOutMin=[]  SumDenOutMax=[]  SumNumOutMin=[]  SumNumOutMax=[]  DivideOutMin=[]  DivideOutMax=[]  UdiffTsProdOutMin=[]  UdiffTsProdOutMax=[]  NTsProdOutMin=[]  NTsProdOutMax=[]  UintegralTsProdOutMin=[]  UintegralTsProdOutMax=[]  UngainTsProdOutMin=[]  UngainTsProdOutMax=[]  IntegratorContinuousStateAttributes=''  IntegratorStateMustResolveToSignalObject=off  IntegratorRTWStateStorageClass=Auto  FilterContinuousStateAttributes=''  FilterStateMustResolveToSignalObject=off  FilterRTWStateStorageClass=Auto  ParallelPVariant=ExternalParameters  IdealPVariant=Disabled  IVariant=ExternalParameters  DVariant=ExternalParameters  IntegratorVariant=Discrete  SatVariant=Disabled  AWVariant=Passthrough  PCopyVariant=Disabled  TRVariant=Disabled  FdbkBlocksVariant=Forward  IdealPFdbkVariant=Disabled  SatFdbkVariant=Disabled  DerivativeFilterVariant=Differentiator  NVariant=Passthrough  NCopyVariant=Disabled_SignalSpec  FilterICVariant=InternalICsDifferentiator  IntegratorICVariant=InternalICs  ExternalResetVariant=Disabled  TRSumVariant=Passthrough  SumFdbkVariant=Disabled  SumVariant=Sum_PID  TsampFilterVariant=InternalTs  TsampNgainVariant=Passthrough  TsampIntegralVariant=Passthrough  ExternalSaturationOutDataTypeStr=Inherit: Same as second input
  stab_yaw_rate_error_calc : Sum  Inputs=|+-
  yaw_cc : Outport
  logging : Outport  Port=2
  wires:
  sys_input/1 -> Bus Selector/1
  Yaw_rate_cmd/1 -> Mux/1, stab_yaw_rate_error_calc/1
  Selector/1 -> stab_yaw_rate_error_calc/2, Mux/2
  Bus Selector/1 -> Selector/1  "<gyro_radps>"
  stab_yaw_rate_error_calc/1 -> stab_yaw_rate_PID/1
  stab_yaw_rate_PID/1 -> Saturation/1
  Demux/1 -> stab_yaw_rate_PID/2
  Demux/2 -> stab_yaw_rate_PID/3
  Demux/3 -> stab_yaw_rate_PID/4
  Mux/1 -> logging/1
  Bus Selector/2 -> Selector1/1  "<param>"
  Selector1/1 -> Demux/1
  Saturation/1 -> yaw_cc/1

== system baseline_queso_1_1/LAND CONTROLLER/Vertical speed controller ==
  sys_data : Inport
  Bus Selector1 : BusSelector  OutputSignals=Navigation Filter Data.ned_pos_m
  Compare To Constant : simulink/Logic and Bit Operations/Compare To Constant  relop=<=  const=Aircraft.Control.land_slow_alt  OutDataTypeStr=boolean
  Constant : Constant  Value=Aircraft.Control.land_speed_fast  OutDataTypeStr=single  SampleTime=framePeriod_s
  Constant1 : Constant  Value=Aircraft.Control.land_speed_slow  OutDataTypeStr=single  SampleTime=framePeriod_s
  Gain : Gain  Gain=-1
  Selector1 : Selector  InputPortWidth=3  IndexOptions=Index vector (dialog)  Indices=[3]  OutputSizes=1
  Switch : Switch  Criteria=u2 > Threshold  Threshold=0.5
  ve_z_cmd_mps : Outport
  wires:
  sys_data/1 -> Bus Selector1/1
  Switch/1 -> ve_z_cmd_mps/1
  Bus Selector1/1 -> Selector1/1  "<ned_pos_m>"
  Selector1/1 -> Gain/1
  Gain/1 -> Compare To Constant/1
  Compare To Constant/1 -> Switch/2
  Constant/1 -> Switch/3
  Constant1/1 -> Switch/1

== system baseline_queso_1_1/LAND CONTROLLER/auto_disarm ==
  note: If altitude is less than slow_land altitude and vertical speed is within 30 cm/s for 10s, system automatically disarm
  sys_input : Inport
  AND : Logic  IconShape=distinctive  AllPortsSameDT=off  OutDataTypeStr=boolean
  Abs : Abs
  Bus Selector : BusSelector  OutputSignals=Navigation Filter Data.ned_pos_m,Navigation Filter Data.ned_vel_mps
  Compare To Constant : simulink/Logic and Bit Operations/Compare To Constant  relop=<=  const=Aircraft.Control.land_slow_alt  OutDataTypeStr=boolean
  Compare To Constant1 : simulink/Logic and Bit Operations/Compare To Constant  relop=<=  const=0.3  OutDataTypeStr=boolean
  Gain : Gain  Gain=-1
  Selector : Selector  InputPortWidth=3  IndexOptions=Index vector (dialog)  Indices=3  OutputSizes=1
  Selector1 : Selector  InputPortWidth=3  IndexOptions=Index vector (dialog)  Indices=3  OutputSizes=1
  disarm motor : Subsystem
  wires:
  sys_input/1 -> Bus Selector/1
  Bus Selector/1 -> Selector/1  "<ned_pos_m>"
  Bus Selector/2 -> Selector1/1  "<ned_vel_mps>"
  Selector/1 -> Gain/1
  Gain/1 -> Compare To Constant/1
  Selector1/1 -> Abs/1
  Abs/1 -> Compare To Constant1/1
  Compare To Constant/1 -> AND/1
  Compare To Constant1/1 -> AND/2
  AND/1 -> disarm motor/Enable

== system baseline_queso_1_1/POS_HOLD CONTROLLER/Horizontal speed controller ==
  note: Assume small roll and pitch angles so translation in Earth frame can be rotated to body frame by rotating by heading only
  sys_input : Inport
  vb_y_cmd_mps : Inport  Port=2
  vb_x_cmd_mps : Inport  Port=3
  2D rotation from NED_xy to body_xy : Subsystem
  Bus Selector : BusSelector  OutputSignals=Navigation Filter Data.heading_rad,Navigation Filter Data.ned_vel_mps
  Demux : Demux  Outputs=2
  Product : Product  Multiplication=Matrix(*)
  Selector : Selector  InputPortWidth=3  IndexOptions=Index vector (dialog)  Indices=[1 2]  OutputSizes=1
  Subsystem : Subsystem
  Subsystem1 : Subsystem
  pitch_angle_cmd_rad : Outport
  roll_angle_cmd_rad : Outport  Port=2
  wires:
  Subsystem1/1(roll_cmd_rad) -> roll_angle_cmd_rad/1  "roll_angle_cmd_rad"
  Subsystem/1(pitch_cmd_rad) -> pitch_angle_cmd_rad/1  "pitch_angle_cmd_rad"
  sys_input/1 -> Bus Selector/1
  Bus Selector/2 -> Selector/1  "<ned_vel_mps>"
  Selector/1 -> Product/2  "ve_xy"
  2D rotation from NED_xy to body_xy/1(2D_rot) -> Product/1
  Product/1 -> Demux/1  "vb_xy"
  Demux/2 -> Subsystem1/2(vb_y)  "vb_y"
  vb_x_cmd_mps/1 -> Subsystem/1(vb_x cmd)  "vb_x cmd"
  Demux/1 -> Subsystem/2(vb_x)  "vb_x"
  Bus Selector/1 -> 2D rotation from NED_xy to body_xy/1(<heading_rad>)  "<heading_rad>"
  vb_y_cmd_mps/1 -> Subsystem1/1(vb_y cmd)

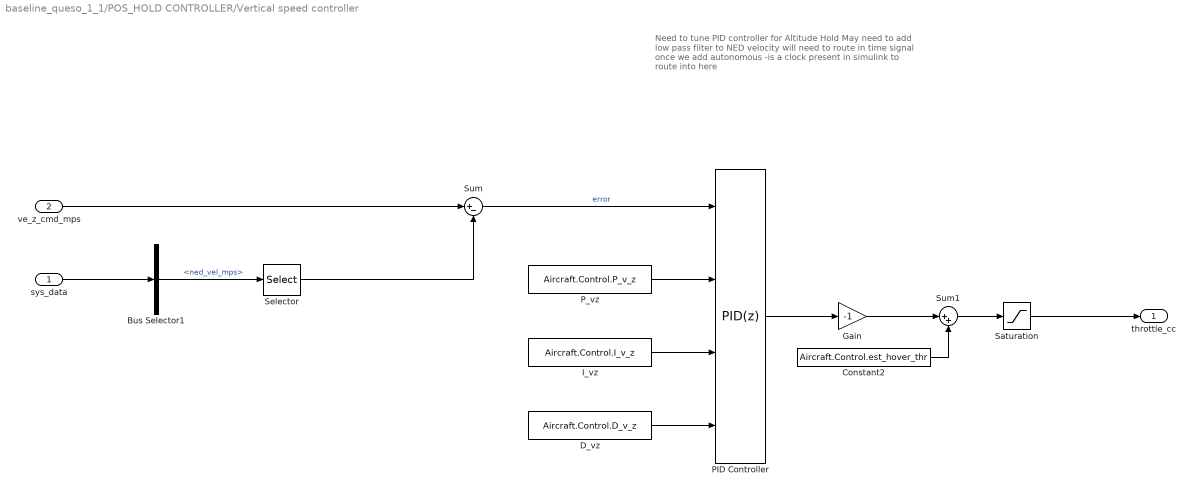
== system baseline_queso_1_1/POS_HOLD CONTROLLER/Vertical speed controller ==
  note: Need to tune PID controller for Altitude Hold
      | May need to add low pass filter to NED velocity
      | will need to route in time signal once we add autonomous
      | -is a clock present in simulink to route into here
  sys_data : Inport
  ve_z_cmd_mps : Inport  Port=2
  Bus Selector1 : BusSelector  OutputSignals=Navigation Filter Data.ned_vel_mps
  Constant2 : Constant  Value=Aircraft.Control.est_hover_thr  OutDataTypeStr=single  SampleTime=framePeriod_s
  D_vz : Constant  Value=Aircraft.Control.D_v_z  OutDataTypeStr=single  SampleTime=framePeriod_s
  Gain : Gain  Gain=-1
  I_vz : Constant  Value=Aircraft.Control.I_v_z  OutDataTypeStr=single  SampleTime=framePeriod_s
  PID Controller : pid_lib/PID Controller  Controller=PID  Form=Parallel  TimeDomain=Discrete-time  UseExternalTs=off  SampleTime=framePeriod_s  IntegratorMethod=Forward Euler  FilterMethod=Forward Euler  ControllerParametersSource=external  P=0  I=0  D=0  UseFilter=off  N=100  TunerSelectOption=Frequency Response Based  InitialConditionSource=internal  InitialConditionForIntegrator=0  InitialConditionForFilter=0  DifferentiatorICPrevScaledInput=0  ExternalReset=none  TrackingMode=off  Kt=1  LimitOutput=off  SatLimitsSource=internal  UpperSaturationLimit=inf  LowerSaturationLimit=-inf  LinearizeAsGain=on  AntiWindupMode=clamping  Kb=1  POutMin=[]  POutMax=[]  IOutMin=[]  IOutMax=[]  DOutMin=[]  DOutMax=[]  NOutMin=[]  NOutMax=[]  SumOutMin=[]  SumOutMax=[]  SaturationOutMin=[]  SaturationOutMax=[]  PParamMin=[]  PParamMax=[]  IParamMin=[]  IParamMax=[]  DParamMin=[]  DParamMax=[]  NParamMin=[]  NParamMax=[]  KbParamMin=[]  KbParamMax=[]  KtParamMin=[]  KtParamMax=[]  KbOutMin=[]  KbOutMax=[]  KtOutMin=[]  KtOutMax=[]  IntegratorOutMin=[]  IntegratorOutMax=[]  FilterOutMin=[]  FilterOutMax=[]  SumI1OutMin=[]  SumI1OutMax=[]  SumI2OutMin=[]  SumI2OutMax=[]  SumI3OutMin=[]  SumI3OutMax=[]  SumI4OutMin=[]  SumI4OutMax=[]  SumDOutMin=[]  SumDOutMax=[]  DifferentiatorOutMin=[]  DifferentiatorOutMax=[]  FilterDiffOutCoefMin=[]  FilterDiffOutCoefMax=[]  ReciprocalOutMin=[]  ReciprocalOutMax=[]  SumDenOutMin=[]  SumDenOutMax=[]  SumNumOutMin=[]  SumNumOutMax=[]  DivideOutMin=[]  DivideOutMax=[]  UdiffTsProdOutMin=[]  UdiffTsProdOutMax=[]  NTsProdOutMin=[]  NTsProdOutMax=[]  UintegralTsProdOutMin=[]  UintegralTsProdOutMax=[]  UngainTsProdOutMin=[]  UngainTsProdOutMax=[]  IntegratorContinuousStateAttributes=''  IntegratorStateMustResolveToSignalObject=off  IntegratorRTWStateStorageClass=Auto  FilterContinuousStateAttributes=''  FilterStateMustResolveToSignalObject=off  FilterRTWStateStorageClass=Auto  ParallelPVariant=ExternalParameters  IdealPVariant=Disabled  IVariant=ExternalParameters  DVariant=ExternalParameters  IntegratorVariant=Discrete  SatVariant=Disabled  AWVariant=Passthrough  PCopyVariant=Disabled  TRVariant=Disabled  FdbkBlocksVariant=Forward  IdealPFdbkVariant=Disabled  SatFdbkVariant=Disabled  DerivativeFilterVariant=Differentiator  NVariant=Passthrough  NCopyVariant=Disabled_SignalSpec  FilterICVariant=InternalICsDifferentiator  IntegratorICVariant=InternalICs  ExternalResetVariant=Disabled  TRSumVariant=Passthrough  SumFdbkVariant=Disabled  SumVariant=Sum_PID  TsampFilterVariant=InternalTs  TsampNgainVariant=Passthrough  TsampIntegralVariant=Passthrough  ExternalSaturationOutDataTypeStr=Inherit: Same as second input
  P_vz : Constant  Value=Aircraft.Control.P_v_z  OutDataTypeStr=single  SampleTime=framePeriod_s
  Saturation : Saturate  UpperLimit=1  LowerLimit=0
  Selector : Selector  InputPortWidth=3  IndexOptions=Index vector (dialog)  Indices=[3]  OutputSizes=1
  Sum : Sum  Inputs=|+-
  Sum1 : Sum  Inputs=|++
  throttle_cc : Outport
  wires:
  Selector/1 -> Sum/2
  D_vz/1 -> PID Controller/4
  Constant2/1 -> Sum1/2
  Sum/1 -> PID Controller/1  "error"
  I_vz/1 -> PID Controller/3
  P_vz/1 -> PID Controller/2
  PID Controller/1 -> Gain/1
  Bus Selector1/1 -> Selector/1  "<ned_vel_mps>"
  Sum1/1 -> Saturation/1
  sys_data/1 -> Bus Selector1/1
  Saturation/1 -> throttle_cc/1
  ve_z_cmd_mps/1 -> Sum/1
  Gain/1 -> Sum1/1

== system baseline_queso_1_1/Pos_Hold_input_conversion/Throttle Mapper ==
  Throttle : Inport
  Compare To Constant : simulink/Logic and Bit Operations/Compare To Constant  relop=<  const=0  OutDataTypeStr=boolean
  Compare To Constant1 : simulink/Logic and Bit Operations/Compare To Constant  relop=>=  const=0  OutDataTypeStr=boolean
  Constant : Constant  Value=Aircraft.Control.v_z_down_max  OutDataTypeStr=single  SampleTime=framePeriod_s
  Constant1 : Constant  Value=Aircraft.Control.v_z_up_max  OutDataTypeStr=single  SampleTime=framePeriod_s
  Double : Constant  Value=2  OutDataTypeStr=single  SampleTime=framePeriod_s
  Gain : Gain  Gain=-1
  Normalize at Zero : Constant  Value=0.5  OutDataTypeStr=single  SampleTime=framePeriod_s
  Product : Product  Inputs=3
  Product1 : Product  Inputs=3
  Sum : Sum  Inputs=|+-
  Sum1 : Sum
  v_z_cmd (-1 to 1) : Product
  Relative Velocity : Outport
  wires:
  Throttle/1 -> Sum/1
  Normalize at Zero/1 -> Sum/2
  Double/1 -> v_z_cmd (-1 to 1)/2
  Sum/1 -> v_z_cmd (-1 to 1)/1
  Sum1/1 -> Gain/1
  v_z_cmd (-1 to 1)/1 -> Product1/2, Compare To Constant1/1, Compare To Constant/1, Product/3
  Constant1/1 -> Product1/3
  Compare To Constant1/1 -> Product1/1
  Product/1 -> Sum1/1
  Product1/1 -> Sum1/2
  Constant/1 -> Product/1
  Compare To Constant/1 -> Product/2
  Gain/1 -> Relative Velocity/1

== system baseline_queso_1_1/Pos_Hold_input_conversion2/Throttle Mapper ==
  Throttle : Inport
  Compare To Constant : simulink/Logic and Bit Operations/Compare To Constant  relop=<  const=0  OutDataTypeStr=boolean
  Compare To Constant1 : simulink/Logic and Bit Operations/Compare To Constant  relop=>=  const=0  OutDataTypeStr=boolean
  Constant : Constant  Value=Aircraft.Control.v_z_down_max  OutDataTypeStr=single
  Constant1 : Constant  Value=Aircraft.Control.v_z_up_max  OutDataTypeStr=single
  Double : Constant  Value=2  OutDataTypeStr=single
  Normalize at Zero : Constant  Value=0.5  OutDataTypeStr=single
  Product : Product  Inputs=3
  Product1 : Product  Inputs=3
  Sum : Sum  Inputs=|+-
  Sum1 : Sum
  v_z_cmd (-1 to 1) : Product
  Relative Velocity : Outport
  wires:
  Throttle/1 -> Sum/1
  Normalize at Zero/1 -> Sum/2
  Double/1 -> v_z_cmd (-1 to 1)/2
  Sum/1 -> v_z_cmd (-1 to 1)/1
  Sum1/1 -> Relative Velocity/1
  v_z_cmd (-1 to 1)/1 -> Product1/2, Compare To Constant1/1, Compare To Constant/1, Product/3
  Constant1/1 -> Product1/3
  Compare To Constant1/1 -> Product1/1
  Product/1 -> Sum1/1
  Product1/1 -> Sum1/2
  Constant/1 -> Product/1
  Compare To Constant/1 -> Product/2
